simulink model "builtin_block_model_PMDC"  (R2023b)
settings: Solver=VariableStepAuto  StartTime=0.0  StopTime=0.5  RelTol=1e-3
values from neighbouring files (symbols this model uses):
  J = 0.00000161    (= 1.61e-06)    [setup_params_pmdc.m]
  Kv = 0.0141    [setup_params_pmdc.m]
  LAA = 0.12    [setup_params_pmdc.m]
  ra = 7    [setup_params_pmdc.m]
  Tl = 0.003    [setup_params_pmdc.m]
  Va = 6    [setup_params_pmdc.m]
libraries: spsControlledVoltageSourceLib x1, spsDCMachineLib x1, sps_lib x1
settings Model: Creator=Noor  LastModifiedBy=USER
settings SolverCC: AlgebraicLoopSolver=TrustRegion
settings DataIOCC: ReturnWorkspaceOutputs=off
settings DebuggingCC: UnconnectedInputMsg=warning  UnconnectedOutputMsg=warning  UnconnectedLineMsg=warning  ArithmeticOperatorsInVariantConditions=warning
settings ModelReferenceCC: EnableRefExpFcnMdlSchedulingChecks=on
settings SFSimCC: SimUseLocalCustomCode=off  CustomCodeUndefinedFunction=UseInterfaceOnly
settings RTWCC: RTWUseLocalCustomCode=off

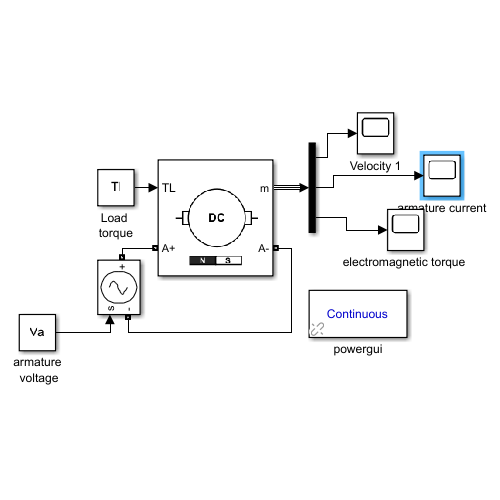
[thumbnail: Simulink's stored preview of the top-level diagram]
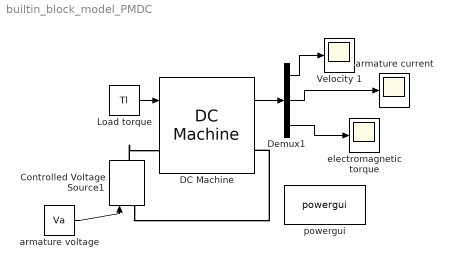
== system builtin_block_model_PMDC ==
  Controlled Voltage Source1 : spsControlledVoltageSourceLib/Controlled Voltage Source  Initialize=off  Source_Type=DC  Amplitude=6  Phase=0  Frequency=0  Measurements=None
  DC Machine : spsDCMachineLib/DC Machine  PresetModel=No  MechanicalLoad=Torque TL  FieldType=Permanent magnet  ShowDetailedParameters=on  MeasurementBus=off  RLa="[ra  LAA]"  RLf="[ 240  120]"  Laf=1.8  MachineConstant=Torque constant (N.m/A)  Ke=Kt  Kt=Kv  J=J  Bm=Bm  Tf=0  w0=1  Ifinit=1  TsPowergui=0  TsBlock=-1
  Demux1 : Demux  Outputs=3
  Load torque : Constant  Value=Tl
  Velocity 1 : Scope
  armature voltage : Constant  Value=Va
  armature current : Scope
  "electromagnetic torque " : Scope
  powergui : sps_lib/powergui  Priority=1  SimulationMode=Continuous  SampleTime=50e-6  frequency=60  Iterations=50  frequencyindice=0  Pbase=100e6  ErrMax=1e-4  UnitsV=kV  UnitsW=MW  buscounter=0  FunctionMessages=off  echomessages=off  EnableUseOfTLC=off  CurrentSourceSwitches=off  DisableSnubberDevices=off  DisableRonSwitches=off  DisableVfSwitches=off  DisplayEquations=off  AutomaticDiscreteSolvers=off  SolverType=Tustin/Backward Euler (TBE)  Interpol=off  ExternalGateDelay=off  methode=off  Ts=100  x0status=blocks  SPID=on  SwTol=0  HookPort=off  NonlinearTolerance=1e-4  nMaxIteration=100  ContinueOnMaxIteration=off  RestoreLinks=warning  ResistiveCurrentMeasurement=off  Frange=[0:2:500]  Ylog=off  Xlog=on  ShowGrid=off  save=off  variable=ZData  structure=0  ZoomFFT=off  StartTime=0.0  cycles=1  DisplayStyle=1  fundamental=60  FreqAxis=off  MaxFrequency=1000  frequencyindicesteady=1  RmsSteady=1  display=off
  wires:
  Demux1/1 -> Velocity 1/1
  Demux1/3 -> "electromagnetic torque "/1
  DC Machine/1 -> Demux1/1
  Demux1/2 -> armature current/1
  Load torque/1 -> DC Machine/1
  armature voltage/1 -> Controlled Voltage Source1/1
  connections:
  Controlled Voltage Source1/RConn1 -- DC Machine/LConn1
  Controlled Voltage Source1/LConn1 -- DC Machine/RConn1
